simulink model "tankModel"  (R2025a)
settings: Solver=VariableStepAuto  StartTime=0.0  StopTime=1000  RelTol=1e-3
values from neighbouring files (symbols this model uses):
  A = 2*pi*r*(r+H)    (= 0.389151343947)    [sizingPrep.m]    (also in sizingSweep.m = result_table.Apogee_m)
  B_liq = 1.2e-3    (= 0.0012)    [sizingPrep.m]
  B_vap = 3.33e-3    (= 0.00333)    [sizingPrep.m]
  C_liq = 0.021    [sizingPrep.m]
  c_p = 0.88    [sizingPrep.m]
  C_vap = 0.021    [sizingPrep.m]
  g = 9.79346    [sizingPrep.m]
  k_liq = 0.109    [sizingPrep.m]
  k_vap = 0.0152    [sizingPrep.m]
  L = 5.0    (= 5)    [PotentialOrificeSize.m]    (also in sizingPrep.m = 0.2032)
  m_tot0 = V_tank*(x_test/py.CoolProp.CoolProp.PropsSI('D', 'T', T, 'Q', 1, 'NitrousOxide') + (1-x_test)/py.CoolProp.CoolProp.PropsSI('D', 'T', T, 'Q', 0, 'NitrousOxide'))^(-1)    [sizingPrep.m]
  mu = 1.825e-5    (= 1.825e-05)    [PotentialOrificeSize.m]    (also in sizingPrep.m = 1.48e-05)
  n_liq = 0.4    [sizingPrep.m]
  n_vap = 0.4    [sizingPrep.m]
  p_amb = 101325    [sizingPrep.m]
  p_fill = 600*6894.76    (= 4136856)    [sizingPrep.m]
  r = 0.08    [runSizingSim.m]    (also in sizingPrep.m = 0.1016; sizingSweep.m; tankEquilibrium.m = 0.1016)
  U_tot0 = ((1-x_test)*py.CoolProp.CoolProp.PropsSI('U', 'T', T, 'Q', 0, 'NitrousOxide')+x_test*py.CoolProp.CoolProp.PropsSI('U', 'T', T, 'Q', 1, 'NitrousOxide'))*m_tot0    [sizingPrep.m]
  V_tank = pi * r^2 * H    (= 0.0164740735604)    [sizingPrep.m]    (also in tankEquilibrium.m = 0.0516128)
  x_full = 0.12    [sizingPrep.m]
libraries: simulink x1
settings Model: Creator=Nick  LastModifiedBy=Pablo

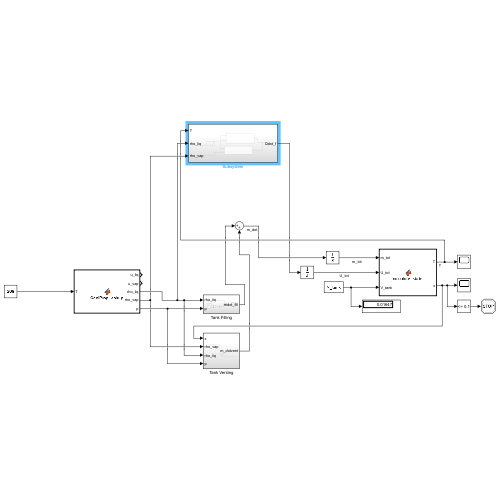
[thumbnail: Simulink's stored preview of the top-level diagram]
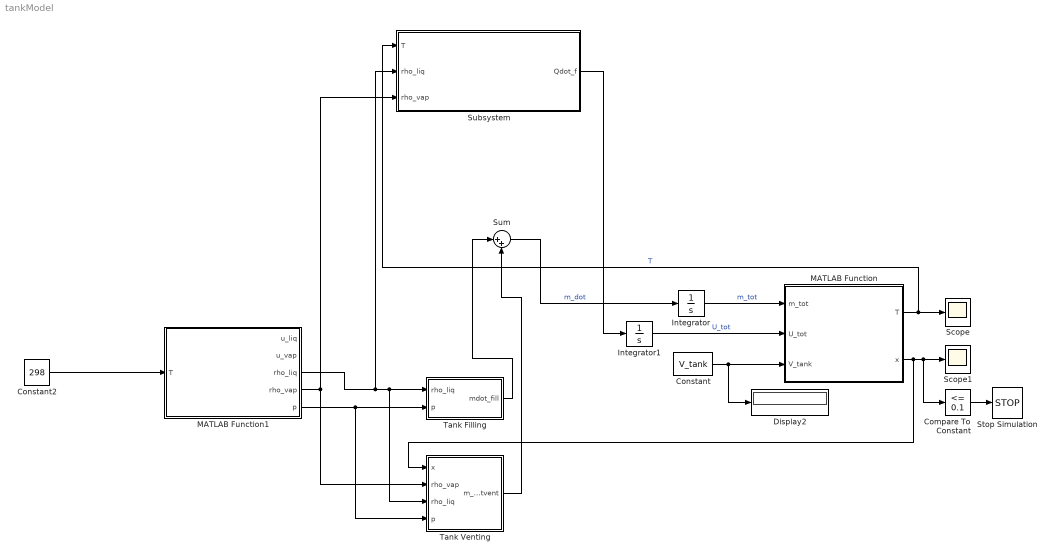
== system tankModel ==
  Compare To Constant : simulink/Logic and Bit Operations/Compare To Constant  relop=<=  const=0.1  OutDataTypeStr=boolean
  Constant : Constant  Value=V_tank
  Constant2 : Constant  Value=298
  Display2 : Display
  Integrator : Integrator  InitialCondition=m_tot0
  Integrator1 : Integrator  InitialCondition=U_tot0
  MATLAB Function : MATLAB Function  TreatAsAtomicUnit=on
  MATLAB Function1 : MATLAB Function  TreatAsAtomicUnit=on
  Scope : Scope
      settings: ActiveDisplayYMinimum=297.58753657496209  ActiveDisplayYMaximum=298.04921593761679
  Scope1 : Scope
      settings: ActiveDisplayYMinimum=-0.012504224387636861  ActiveDisplayYMaximum=1.1125380194909855
  Stop Simulation : Stop
  Subsystem : Subsystem
  Sum : Sum  Inputs=|++
  Tank Filling : Subsystem
  Tank Venting : Subsystem
  wires:
  MATLAB Function/2(x) -> Tank Venting/1(x), Scope1/1, Compare To Constant/1
  Constant/1 -> Display2/1, MATLAB Function/3(V_tank)
  Compare To Constant/1 -> Stop Simulation/1
  Integrator/1 -> MATLAB Function/1(m_tot)  "m_tot"
  Integrator1/1 -> MATLAB Function/2(U_tot)  "U_tot"
  MATLAB Function/1(T) -> Scope/1, Subsystem/1(T)  "T"
  Constant2/1 -> MATLAB Function1/1(T)
  Tank Filling/1(mdot_fill) -> Sum/1
  MATLAB Function1/3(rho_liq) -> Subsystem/2(rho_liq), Tank Venting/3(rho_liq), Tank Filling/1(rho_liq)
  MATLAB Function1/5(p) -> Tank Venting/4(p), Tank Filling/2(p)
  Sum/1 -> Integrator/1  "m_dot"
  MATLAB Function1/4(rho_vap) -> Subsystem/3(rho_vap), Tank Venting/2(rho_vap)
  Tank Venting/1(m_dotvent) -> Sum/2
  Subsystem/1(Qdot_f) -> Integrator1/1

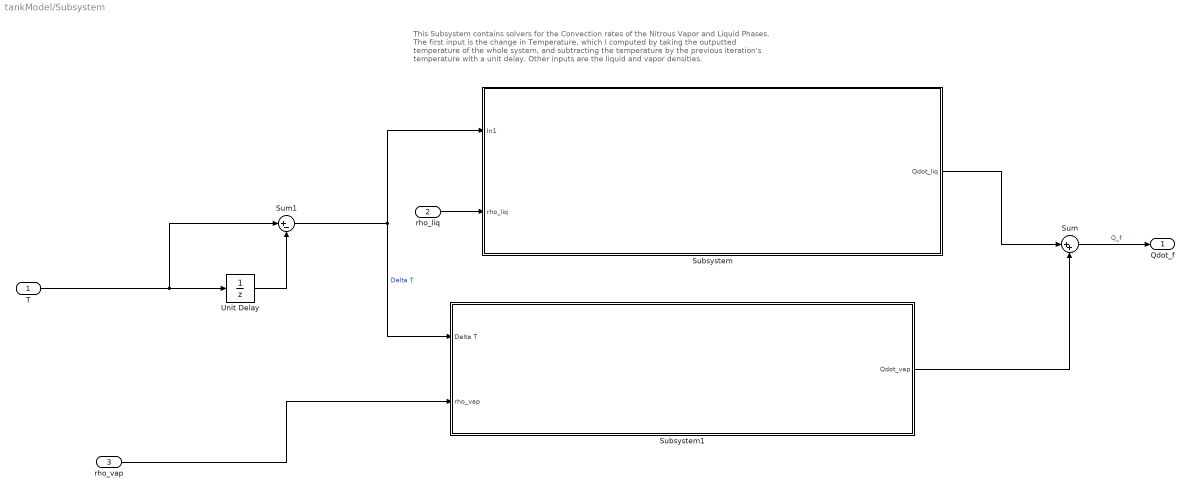
== system tankModel/Subsystem ==
  note: This Subsystem contains solvers for the Convection rates of the Nitrous Vapor and Liquid Phases. The first input is the change in Temperature, which I computed by taking the outputted temperature of the whole system, and subtracting the temperature by the previous iteration's temperature with a unit delay. Other inputs are the liquid and vapor densities.
  T : Inport
  rho_liq : Inport  Port=2
  rho_vap : Inport  Port=3
  Subsystem : Subsystem
  Subsystem1 : Subsystem
  Sum : Sum  Inputs=|++
  Sum1 : Sum  Inputs=|+-
  Unit Delay : UnitDelay  SampleTime=-1  HasFrameUpgradeWarning=on
  Qdot_f : Outport
  wires:
  Unit Delay/1 -> Sum1/2
  T/1 -> Sum1/1, Unit Delay/1
  Sum1/1 -> Subsystem1/1(Delta T), Subsystem/1(In1)  "Delta T"
  rho_liq/1 -> Subsystem/2(rho_liq)
  Subsystem/1(Qdot_liq) -> Sum/1
  rho_vap/1 -> Subsystem1/2(rho_vap)
  Subsystem1/1(Qdot_vap) -> Sum/2
  Sum/1 -> Qdot_f/1  "Q_f"

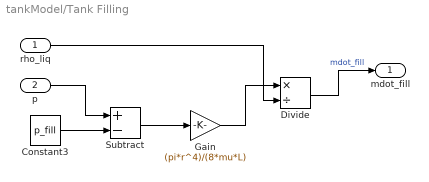
== system tankModel/Tank Filling ==
  rho_liq : Inport
  p : Inport  Port=2
  Constant3 : Constant  Value=p_fill
  Divide : Product  Inputs=*/
  Gain : Gain  Gain=(pi*r^4)/(8*mu*L)
  Subtract : Sum  Inputs=+-
  mdot_fill : Outport
  wires:
  Divide/1 -> mdot_fill/1  "mdot_fill"
  Subtract/1 -> Gain/1
  Constant3/1 -> Subtract/2
  rho_liq/1 -> Divide/2
  Gain/1 -> Divide/1
  p/1 -> Subtract/1

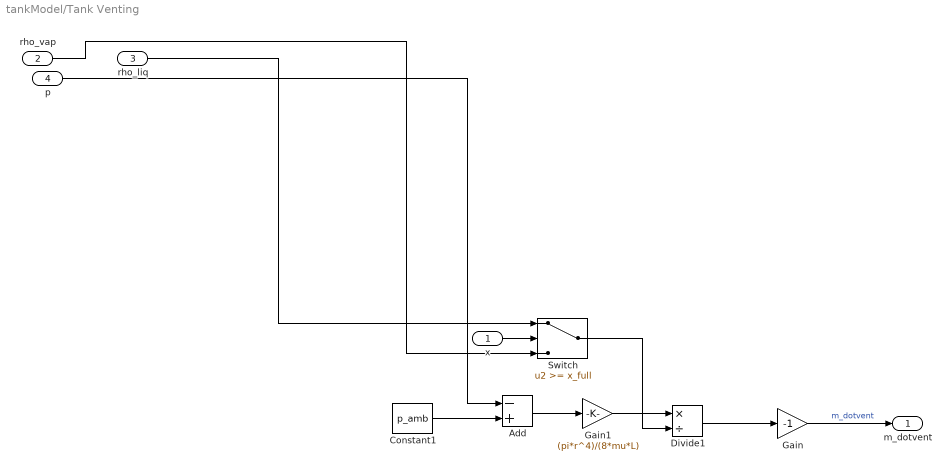
== system tankModel/Tank Venting ==
  x : Inport
  rho_vap : Inport  Port=2
  rho_liq : Inport  Port=3
  p : Inport  Port=4
  Add : Sum  Inputs=-+
  Constant1 : Constant  Value=p_amb
  Divide1 : Product  Inputs=*/
  Gain : Gain  Gain=-1
  Gain1 : Gain  Gain=(pi*r^4)/(8*mu*L)
  Switch : Switch  Threshold=x_full  SaturateOnIntegerOverflow=off  InputSameDT=off
  m_dotvent : Outport
  wires:
  Add/1 -> Gain1/1
  Switch/1 -> Divide1/2
  Gain1/1 -> Divide1/1
  Divide1/1 -> Gain/1
  p/1 -> Add/1
  Constant1/1 -> Add/2
  x/1 -> Switch/2
  rho_liq/1 -> Switch/1
  rho_vap/1 -> Switch/3
  Gain/1 -> m_dotvent/1  "m_dotvent"

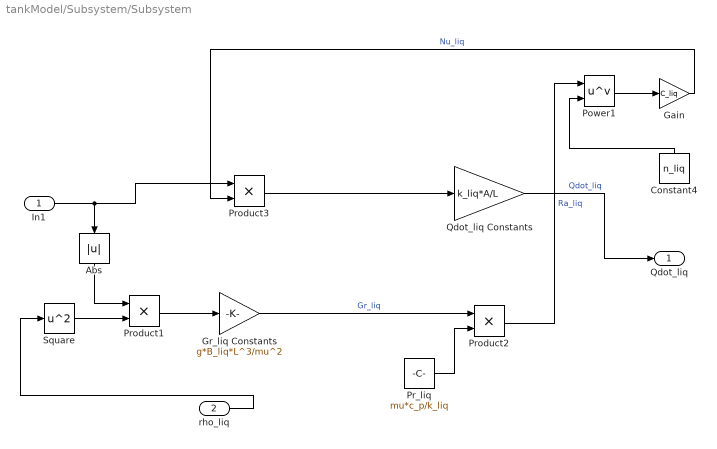
== system tankModel/Subsystem/Subsystem ==
  In1 : Inport
  rho_liq : Inport  Port=2
  Abs : Abs  SaturateOnIntegerOverflow=off
  Constant4 : Constant  Value=n_liq
  Gain : Gain  Gain=C_liq
  Gr_liq Constants : Gain  Gain=g*B_liq*L^3/mu^2
  Power1 : Math  Operator=pow
  Pr_liq : Constant  Value=mu*c_p/k_liq
  Product1 : Product
  Product2 : Product
  Product3 : Product
  Qdot_liq Constants : Gain  Gain=k_liq*A/L
  Square : Math  Operator=square
  Qdot_liq : Outport
  wires:
  Qdot_liq Constants/1 -> Qdot_liq/1  "Qdot_liq"
  Product2/1 -> Power1/1  "Ra_liq"
  Pr_liq/1 -> Product2/2
  In1/1 -> Product3/1, Abs/1
  Gain/1 -> Product3/2  "Nu_liq"
  Gr_liq Constants/1 -> Product2/1  "Gr_liq"
  Product1/1 -> Gr_liq Constants/1
  Square/1 -> Product1/2
  Power1/1 -> Gain/1
  rho_liq/1 -> Square/1
  Constant4/1 -> Power1/2
  Product3/1 -> Qdot_liq Constants/1
  Abs/1 -> Product1/1

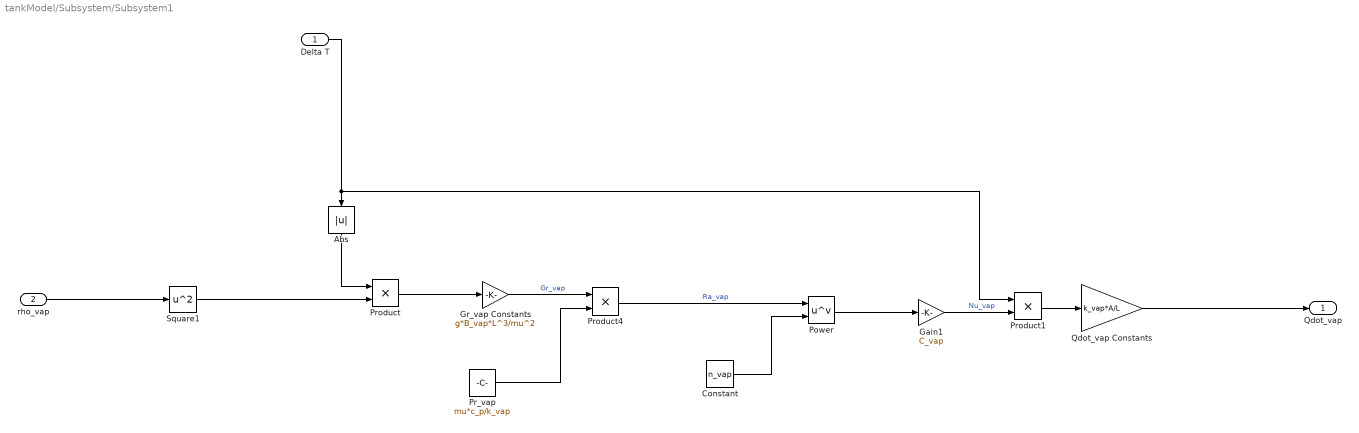
== system tankModel/Subsystem/Subsystem1 ==
  Delta T : Inport
  rho_vap : Inport  Port=2
  Abs : Abs  SaturateOnIntegerOverflow=off
  Constant : Constant  Value=n_vap
  Gain1 : Gain  Gain=C_vap
  Gr_vap Constants : Gain  Gain=g*B_vap*L^3/mu^2
  Power : Math  Operator=pow
  Pr_vap : Constant  Value=mu*c_p/k_vap
  Product : Product
  Product1 : Product
  Product4 : Product
  Qdot_vap Constants : Gain  Gain=k_vap*A/L
  Square1 : Math  Operator=square
  Qdot_vap : Outport
  wires:
  rho_vap/1 -> Square1/1
  Qdot_vap Constants/1 -> Qdot_vap/1
  Gain1/1 -> Product1/2  "Nu_vap"
  Square1/1 -> Product/2
  Abs/1 -> Product/1
  Delta T/1 -> Product1/1, Abs/1
  Product4/1 -> Power/1  "Ra_vap"
  Pr_vap/1 -> Product4/2
  Power/1 -> Gain1/1
  Product1/1 -> Qdot_vap Constants/1
  Constant/1 -> Power/2
  Product/1 -> Gr_vap Constants/1
  Gr_vap Constants/1 -> Product4/1  "Gr_vap"

== matlab function tankModel/MATLAB Function1 ==
  data: T input; u_liq output; u_vap output; rho_liq output; rho_vap output; p output
function [u_liq,u_vap,rho_liq,rho_vap,p] = CoolPropLookup(T)
lookup = load('CoolPropLookup.mat');
u_liq = interp1(lookup.T_range, lookup.u_liq, T,"linear");
u_vap = interp1(lookup.T_range, lookup.u_vap, T,"linear");
rho_liq = interp1(lookup.T_range, lookup.rho_liq, T,"linear");
rho_vap = interp1(lookup.T_range, lookup.rho_vap, T,"linear");
p = interp1(lookup.T_range, lookup.p, T, "linear");

== matlab function tankModel/MATLAB Function ==
  data: m_tot input; T output; U_tot input; V_tank input; x output
function [T, x]= calculate_state(m_tot, U_tot, V_tank)
    lookup = load('CoolPropLookup.mat');
    % Resduals anonymous function given U_tot m_tot and V_tank
    residual_function = @(x) [(1-x(1)) * interp1(lookup.T_range, lookup.u_liq, x(2), "linear") + x(1) * interp1(lookup.T_range, lookup.u_vap, x(2), "linear")-U_tot/m_tot;
             (x(1)/interp1(lookup.T_range, lookup.rho_vap, x(2), "linear") + (1-x(1))/interp1(lookup.T_range, lookup.rho_liq, x(2), "linear"))*m_tot-V_tank];
    % Innitial guess
    x0 = [0.5; 298];
    % solve
    options = optimoptions('fsolve', 'Algorithm', 'levenberg-marquardt', 'Display', 'iter');
    [solution,fval] = fsolve(residual_function,x0,options);
    x = solution(1);
    T = solution(2);
